simulink model "rectifier_24pulse"  (R2014a)
settings: Solver=VariableStepDiscrete  StartTime=0.0  StopTime=0.2  FixedStep=Ts  MaxStep=1e-4  RelTol=1e-4
PreLoadFcn:
  | Ts = 5e-6;
InitFcn:
  | Ts = 5e-6;
StartFcn:
  | tic;
StopFcn:
  | toc;
undefined symbols (not defined in the file or in its folder): C
libraries: powerlib x16
settings Model: Creator=gdudgeon  LastModifiedBy=cosorio
settings DataIOCC: SignalLoggingSaveFormat=ModelDataLogs  SaveTime=off
settings OptimizationCC: ExpressionDepthLimit=2147483647  InitFltsAndDblsToZero=on
settings DebuggingCC: SaveWithParameterizedLinksMsg=none  UnderspecifiedInitializationDetection=Classic  SignalResolutionControl=TryResolveAllWithWarning  SolverPrmCheckMsg=none  MultiTaskDSMMsg=warning  MultiTaskCondExecSysMsg=none  FcnCallInpInsideContextMsg=UseLocalSettings  StateNameClashWarn=warning
settings RTWCC: IncludeERTFirstTime=on
settings GRTTargetCC: TargetFcnLib=ansi_tfl_tmw.mat  CombineOutputUpdateFcns=off  GRTInterface=on

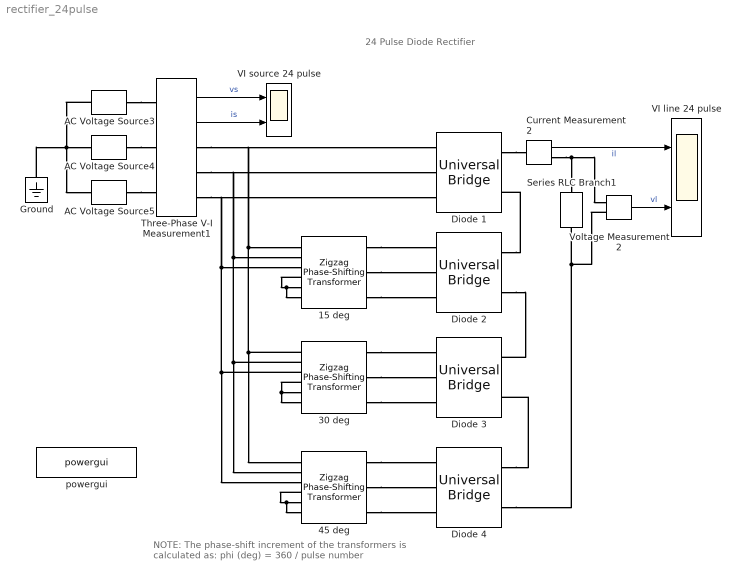
== system rectifier_24pulse ==
  note: NOTE: The phase-shift
      | increment of the transformers
      | is calculated as:
      | phi (deg) = 360 / pulse number
  note: 24 Pulse Diode Rectifier
  15 deg : powerlib/Elements/Zigzag Phase-Shifting Transformer  SecondaryConnection=Y  UNITS=pu  NominalPower=[ 1e4 60 ]  PrimaryVoltage=100/sqrt(2)  SecondaryVoltage="[ 100/sqrt(2)  15 ]"  Winding1=[ 1e-5 1e-5 ]  Winding2=[ 1e-5 1e-5 ]  Winding3=[ 1e-5 1e-5 ]  SetSaturation=off  RmLm=[ 500 500 ]  Rm=500  Saturation=[ 0,0 ; 0.0024,1.2 ; 1.0,1.52 ]  SetInitialFlux=off  Measurements=None  InitialFluxes=[0,0,0]  MoreParameters=on  BreakLoop=off  DataType=off
  30 deg : powerlib/Elements/Zigzag Phase-Shifting Transformer  SecondaryConnection=Y  UNITS=pu  NominalPower=[ 1e4 60 ]  PrimaryVoltage=100/sqrt(2)  SecondaryVoltage="[ 100/sqrt(2)  30 ]"  Winding1=[ 1e-5 1e-5 ]  Winding2=[ 1e-5 1e-5 ]  Winding3=[ 1e-5 1e-5 ]  SetSaturation=off  RmLm=[ 500 500 ]  Rm=500  Saturation=[ 0,0 ; 0.0024,1.2 ; 1.0,1.52 ]  SetInitialFlux=off  Measurements=None  InitialFluxes=[0,0,0]  MoreParameters=on  BreakLoop=off  DataType=off
  45 deg : powerlib/Elements/Zigzag Phase-Shifting Transformer  SecondaryConnection=Y  UNITS=pu  NominalPower=[ 1e4 60 ]  PrimaryVoltage=100/sqrt(2)  SecondaryVoltage="[ 100/sqrt(2)  45 ]"  Winding1=[ 1e-5 1e-5 ]  Winding2=[ 1e-5 1e-5 ]  Winding3=[ 1e-5 1e-5 ]  SetSaturation=off  RmLm=[ 500 500 ]  Rm=500  Saturation=[ 0,0 ; 0.0024,1.2 ; 1.0,1.52 ]  SetInitialFlux=off  Measurements=None  InitialFluxes=[0,0,0]  MoreParameters=on  BreakLoop=off  DataType=off
  AC Voltage Source3 : powerlib/Electrical Sources/AC Voltage Source  Amplitude=100/sqrt(3)  Phase=0  Frequency=60  SampleTime=0  Measurements=None
  AC Voltage Source4 : powerlib/Electrical Sources/AC Voltage Source  Amplitude=100/sqrt(3)  Phase=-120  Frequency=60  SampleTime=0  Measurements=None
  AC Voltage Source5 : powerlib/Electrical Sources/AC Voltage Source  Amplitude=100/sqrt(3)  Phase=120  Frequency=60  SampleTime=0  Measurements=None
  Current Measurement2 : powerlib/Measurements/Current Measurement  PhasorSimulation=off  OutputType=Complex  PSBequivalent=0
  Diode {1..4} (4 alike) : powerlib/Power Electronics/Universal Bridge  Arms=3  SnubberResistance=1000  SnubberCapacitance=1e-6  Device=Diodes  Ron=1e-3  Lon=0  ForwardVoltages=[0 0]  ForwardVoltage=0.8  GTOparameters=[0 0]  IGBTparameters=[1e-6 2e-6]  Measurements=None  Measurements_2=None  converterType=Rectifier
  Ground : powerlib/Elements/Ground  LConnTagsString=a
  Series RLC Branch1 : powerlib/Elements/Series RLC Branch  LConnTagsString=__new0  RConnTagsString=__new0  BranchType=R  Resistance=1  Inductance=[]  SetiL0=off  InitialCurrent=0  Capacitance=C  Setx0=off  InitialVoltage=0  Measurements=None
  Three-Phase V-I Measurement1 : powerlib/Measurements/Three-Phase V-I Measurement  VoltageMeasurement=phase-to-phase  SetLabelV=off  LabelV=Vabc  Vpu=off  VpuLL=off  CurrentMeasurement=yes  SetLabelI=off  LabelI=Iabc  Ipu=off  Pbase=100e6  Vbase=500e3  OutputType=Complex  PhasorSimulation=off  PSBequivalent=0
  VI line 24 pulse : Scope  NumInputPorts=2
      settings: YMin=0~0  YMax=500~500  SaveName=viline24
  VI source 24 pulse : Scope  NumInputPorts=2
      settings: YMin=-200~-2000  YMax=200~2000  SaveName=visource24
  Voltage Measurement2 : powerlib/Measurements/Voltage Measurement  PhasorSimulation=off  OutputType=Complex  PSBequivalent=0
  powergui : powerlib/powergui  Priority=2  SimulationMode=Discrete  SolverType=Tustin  SampleTime=Ts  frequency=60  SPID=off  DisableSnubberDevices=off  DisableRonSwitches=off  DisableVfSwitches=off  SwTol=0  Interpol=off  DisplayEquations=off  Ts=0  methode=off  frequencyindice=60  Pbase=100e6  ErrMax=1e-4  Iterations=50  UnitsV=kV  UnitsW=MW  FunctionMessages=off  echomessages=off  HookPort=off  EnableUseOfTLC=off  x0status=blocks  RestoreLinks=warning  ResistiveCurrentMeasurement=off  Frange=[0:2:500]  Ylog=off  Xlog=on  ShowGrid=off  save=off  variable=ZData  structure=visource24  ZoomFFT=off  StartTime=0.05  cycles=5  DisplayStyle=1  fundamental=60  FreqAxis=on  MaxFrequency=4000  frequencyindicesteady=1  RmsSteady=1  display=off
  wires:
  Three-Phase V-I Measurement1/1 -> VI source 24 pulse/1  "vs"
  Three-Phase V-I Measurement1/2 -> VI source 24 pulse/2  "is"
  Voltage Measurement2/1 -> VI line 24 pulse/2  "vl"
  Current Measurement2/1 -> VI line 24 pulse/1  "il"
  connections:
  30 deg/LConn1 -- 45 deg/LConn1 -- 15 deg/LConn1 -- Diode 1/LConn1 -- Three-Phase V-I Measurement1/RConn1
  30 deg/LConn2 -- 45 deg/LConn2 -- 15 deg/LConn2 -- Diode 1/LConn2 -- Three-Phase V-I Measurement1/RConn2
  30 deg/LConn3 -- 45 deg/LConn3 -- 15 deg/LConn3 -- Diode 1/LConn3 -- Three-Phase V-I Measurement1/RConn3
  Current Measurement2/RConn1 -- Voltage Measurement2/LConn1 -- Series RLC Branch1/LConn1
  Voltage Measurement2/LConn2 -- Diode 4/RConn2 -- Series RLC Branch1/RConn1
  Diode 1/RConn1 -- Current Measurement2/LConn1
  AC Voltage Source5/RConn1 -- Three-Phase V-I Measurement1/LConn3
  AC Voltage Source3/RConn1 -- Three-Phase V-I Measurement1/LConn1
  AC Voltage Source4/RConn1 -- Three-Phase V-I Measurement1/LConn2
  30 deg/RConn1 -- Diode 3/LConn1
  30 deg/RConn2 -- Diode 3/LConn2
  30 deg/RConn3 -- Diode 3/LConn3
  Diode 2/RConn2 -- Diode 3/RConn1
  15 deg/RConn3 -- Diode 2/LConn3
  15 deg/RConn2 -- Diode 2/LConn2
  15 deg/RConn1 -- Diode 2/LConn1
  Diode 2/RConn1 -- Diode 1/RConn2
  45 deg/RConn1 -- Diode 4/LConn1
  45 deg/RConn2 -- Diode 4/LConn2
  45 deg/RConn3 -- Diode 4/LConn3
  Diode 4/RConn1 -- Diode 3/RConn2
  AC Voltage Source3/LConn1 -- Ground/LConn1 -- AC Voltage Source5/LConn1 -- AC Voltage Source4/LConn1
  45 deg/LConn5 -- 45 deg/LConn4 -- 45 deg/LConn6
  30 deg/LConn4 -- 30 deg/LConn6 -- 30 deg/LConn5
  15 deg/LConn5 -- 15 deg/LConn4 -- 15 deg/LConn6
